simulink model "Copy_of_modello_completo_2_12"  (R2020b)
settings: Solver=FixedStepDiscrete  StartTime=0.0  StopTime=Inf  FixedStep=0.02  RelTol=1e-3  EnableMultiTasking=on
undefined symbols (not defined in the file or in its folder): attuatore_Amax, attuatore_Amin, attuatore_Emax, attuatore_Emin, attuatore_Rmax, attuatore_Rmin, attuatore_Tmax, attuatore_Tmin, DiscIntNeverNeededParam, interventoA_05, interventoA_1, interventoE_05, interventoE_1, interventoT, inv_A, inv_comp_h, inv_E, inv_R, inv_T, K_AW_B_AP_quota, K_AW_B_becc, K_AW_B_imb, K_AW_B_roll, K_imb_inv, Kd_h_app, Kd_h_flare, Ki_AP_quota_select, Ki_AP_rotta, Ki_AP_vel, Ki_becch, Ki_h_app, Ki_h_cruise, Ki_h_flare, Ki_roll, Kp_AP_quota_hold_h, Kp_AP_quota_hold_l, Kp_AP_quota_select, Kp_AP_rotta, Kp_AP_vel, Kp_becch, Kp_comp_h, Kp_h_app_max, Kp_h_app_min, Kp_h_cruise, Kp_h_flare, Kp_imb, Kp_p, Kp_q, Kp_roll, Kp_Rotta_ATO, Newton, phi_max, phi_min, Raphson, safe_phi, safe_V, t_AP, theta_max, theta_min, time_alarm_SAFE ... (+5)
libraries: simulink_extras x41, arduinolib x26, pid_lib x8, svdutilitieslib x6, simulink x3, dspsigops x3, aerolibtransform2sys x2, aerolibtransform2 x2, cstblocks x1
(part 6 of 8)

== stateflow chart Copy_of_modello_completo_2_12/AUTOPILOTA/Subsystem1/Subsystem1/Chart1 ==
  state Allignment1
    du:
    maneuver_selector=1;
    landing_selector=0;
    trig_approach = 0;
    trig_flare = 0;
    approach_selector = 0;
  state Abort
    du:
    maneuver_selector=1;
    landing_selector=0;
    trig_approach = 0;
    trig_flare = 0;
    approach_selector = 0;
  state Allignment
    du:
    trig_flare = 0;
    approach_selector = 0;
    maneuver_selector=1;
    landing_selector=0;
    trig_approach = 0;
  state Approach
    du:
    trig_flare = 0;
    trig_approach = 1;
    approach_selector = 1;
    landing_selector=1;
    maneuver_selector=2;
  state Flare
    du:
    trig_approach = 0;
    trig_flare = 1;
    approach_selector = 0;
    landing_selector=2;
    maneuver_selector=3;
  (default) -> Allignment1 : {maneuver_selector=1;
      |  landing_selector=0;
      |  trig_approach = 0;
      |  trig_flare = 0;
      |  approach_selector = 1;}
  Approach -> Allignment1 [order 2] : [modo ~= 4]
  Flare -> Allignment1 [order 2] : [modo ~= 4]
  Allignment -> Allignment1 [order 2] : [modo ~= 4]
  Approach -> Abort [order 3] : [landing_abort == 1]
  Allignment -> Approach [order 1] : [(h > 35) && (h < 60) && (dist <= h*(1/tan(3*pi/180))+100) && (dist >= h*(1/tan(4*pi/180))+100) && (counter >1)]
  Allignment1 -> Allignment : [modo == 4]
  Approach -> Flare [order 1] : [ (x_e >= x_f) && ((h <= (h_f + 1.5)) ||( h > (h_f - 1)))]
  Flare -> (junction 67) [order 1] : [TAS < 3]{landing_selector=0;}
  data: h input; dist input; counter input; maneuver_selector output; x_e input; x_f input; h_f input; TAS input; landing_selector output; trig_approach output; modo input; trig_flare output; approach_selector output; landing_abort input

== matlab function Copy_of_modello_completo_2_12/AIR TX/Heartbeat/Alarm set ==
  data: Alarm input; H_mav output; Rx_mode input

%%

function H_mav = Allarm_set(Alarm, Rx_mode)
%#cambia lo stato se c'è un allarme attivo
% Allarm: possibili allarmi proveniente dall'autopilota
% Rx_mode: richiesta da parte della stazione di terra
% H_mav: setto i parametri Base_mode e System_status del Heartbeat


H_mav = uint8(Rx_mode); % setta la modalità con quella ricevuta da terra

% se un allarme si attiva ha la precedenza sulla richiesta della QGC

if Alarm(1) == 1 % ovvero l'aereo è entrato in safe e si pone su traettoria circolare di sicurezza
    
    H_mav(1) = uint8(220); % MAV_MODE_AUTO_ARMED
    H_mav(2) = uint8(5);   % MAV_STATE_CRITICAL
%     H_mav(3) = uint8(128); % MAV_MODE_FLAG_SAFETY_ARMED

end

% se l'allareme di intervento pilota è attivo ha precedenza sull'allarm
% sefe per cui bisogna riscrivere lo stato del pilota

if Alarm(2) == 1 % si è attivato l'allarme dell'intervento pilota 
    
    H_mav(1) = uint8(216); % MAV_MODE_GUIDED_ARMED
    H_mav(2) = uint8(4);   % MAV_STATE_ACTIVE
%     H_mav(3) = uint8(8);   % MAV_MODE_FLAG_GUIDED_ENABLED

end

== matlab function Copy_of_modello_completo_2_12/AIR TX/If_subsystem/iflogic_function ==
  data: H50 input; iflogic output; H10 input
function iflogic = fcn(H50,H10)
%#codegen
% prende in ingeresso i counter che contano il tempo
% e dice quale messaggio bisogna inviare in base alle frequenze scelte in
% Heartbeat:            1Hz
% SCALED_IMU:           20Hz
%attitude:              20Hz
%GLOBAL_POSITION_INT:   1Hz
%SYS_STATUS:            3Hz
%VFR_HUD:               2Hz
%SERVO_OUTPUT_RAW       1Hz
%SCALED_PRESSURE        1Hz

if H50 == 1  || H50==3
    iflogic=uint8(26); % SCALED_IMU 20Hz
elseif H50==2 || H50==4
    iflogic=uint8(30); %attitude 20Hz
elseif  H50==0 && H10==2
    iflogic=uint8(33); %GLOBAL_POSITION_INT 1Hz
elseif  H50==0 && H10==6
    iflogic=uint8(34); %GLOBAL_POSITION_INT_RAW 1Hz
elseif  H50==0 && H10==0
    iflogic=uint8(0); %Heartbeat 1Hz
elseif H50==0 && (H10==1 || H10==5 || H10==9)
    iflogic=uint8(1); %SYS_STATUS 3Hz
elseif H50==0 && (H10==3 || H10==8)
    iflogic=uint8(74); %VFR_HUD 2Hz
elseif H50==0 && (H10==7)
    iflogic=uint8(36); %SERVO_OUTPUT_RAW 1Hz
elseif H50==0 && (H10==4)
    iflogic=uint8(29); %SCALED_PRESSURE 1Hz
else
    iflogic=uint8(255); %non esiste nessun messaggio con questo codice
    
end

== matlab function Copy_of_modello_completo_2_12/AIR TX/Waypoints/MATLAB Function ==
  data: WP_info_in input; WP_param_in input; WP_info output; GC_info input; WP_param output
function [WP_info,WP_param] = fcn(WP_info_in,WP_param_in, GC_info)
%#codegen
WP_info=WP_info_in(1,:); %%per sicurezza
WP_param=WP_param_in(1,:); %%per sicurezza
[m,n]=size(WP_info_in);
if GC_info(1)==2
    if GC_info(2)>=0 && GC_info(2)<m %per poter inviare i MISSION_ITEM
        WP_info=WP_info_in(GC_info(2)+1,:);
        WP_param=WP_param_in(GC_info(2)+1,:);
    end
end
if GC_info(1)==3 && GC_info(2)>=0 && GC_info(2)<200 %per poter inviae i MISSION_REQUEST
    WP_info=WP_info_in(GC_info(2)+1,:);
end

== matlab function Copy_of_modello_completo_2_12/AUTOPILOTA/Subsystem1/Subsystem/VETTORIALE ==
  data: V_vett output double; h_vett output double; rotta_vett output double; RC_vett output double; ingaggio_AP_mem output; modo input; IAS input; ALT input; HDG input; I_RC input; ingaggio_AP input; ROTTA input; VELOCITA input; QUOTA input; RC input; HEADING input; TAS input; h input; RC_default input; ingaggio_AP_pre input uint8; modo_pre input; IAS_pre input uint8; ALT_pre input uint8; HDG_pre input uint8; modo_pre_mem output; IAS_pre_mem output uint8; ALT_pre_mem output uint8; HDG_pre_mem output uint8
function [V_vett, h_vett, rotta_vett, RC_vett, ingaggio_AP_mem, modo_pre_mem, IAS_pre_mem, ALT_pre_mem, HDG_pre_mem] = vettoriale(modo, IAS, ALT, HDG, I_RC, ingaggio_AP ,ROTTA, VELOCITA, QUOTA, RC, HEADING, TAS, h, RC_default, ingaggio_AP_pre,modo_pre, IAS_pre, ALT_pre, HDG_pre)
%#codegen

persistent V_ref ALT_ref HDG_ref

if isempty(V_ref)
    
    V_ref = 0;
    
end

if isempty(ALT_ref)
    
    ALT_ref = 0;
    
end

if isempty(HDG_ref)
    
    HDG_ref = 0;
    
end

if (ingaggio_AP ~= ingaggio_AP_pre || modo ~= modo_pre || IAS ~= IAS_pre)
    
    V_ref = TAS;
    
end

if (ingaggio_AP ~= ingaggio_AP_pre || modo ~= modo_pre || ALT ~= ALT_pre)
    
    ALT_ref = h;
    
end

if (ingaggio_AP ~= ingaggio_AP_pre || modo ~= modo_pre || HDG ~= HDG_pre)
    
    HDG_ref = HEADING;
    
end

if (IAS == 1)
    
    V_vett = VELOCITA;
    
else
    
    V_vett = V_ref;
    
end

if (ALT == 1)
    
    h_vett = QUOTA;
    
else
    
   h_vett = ALT_ref;
    
end

if (HDG == 1)
    
    rotta_vett = ROTTA;
    
else
    
  rotta_vett = HDG_ref;
    
end

RC_vett = 0;

if ((h_vett - h) >= 0) 
    
    if (I_RC == 1)
    
        RC_vett = RC;
    
    else
    
        RC_vett = RC_default;
    
    end
    
elseif ((h_vett - h) < 0 ) 
    
    if (I_RC == 1)
    
        RC_vett = -RC;
    
    else
    
        RC_vett = -RC_default;
    
    end 
    
end
    
ingaggio_AP_mem = uint8(ingaggio_AP);
modo_pre_mem = modo;
IAS_pre_mem  = uint8(IAS);
ALT_pre_mem  = uint8(ALT);
HDG_pre_mem  = uint8(HDG);

== matlab function Copy_of_modello_completo_2_12/Misure Sensori/BMP_280/MATLAB Function1 ==
  data: T_0 input; P_ref input; h_ output; P input
function h_  = fcn( T_0, P_ref,P)
%#codegen

g     = 9.81;    %accelerazione di gravità
R_gas = 287.05;  %costante dei gas perfetti
dTdh  = -0.0065; %gradiente termico verticale in atmosfera standard 

T_0        = T_0+273.15;


    
h_= ((R_gas/g)*log(P_ref/P)*T_0)/(1-(dTdh*0.5*(R_gas/g)*log(P_ref/P)));

== matlab function Copy_of_modello_completo_2_12/AIR RX/MATLAB Function1 ==
  data: Base_mode input; GC_req input; value_c input; WP_info_in input; WP_param_in input; mem_out input; T_number input; T_ref input; Mav_state input; AP_int output; AP_rif output; H_mav output; SyS_data output; GC_info output; WP_db_out output; WP_db_param output; WP_AL output; Val_out_MAV output; T_0 output; AP_int_mem input; Base_mode_to_SF output; test output
function [AP_int, AP_rif, H_mav, SyS_data, GC_info, WP_db_out, WP_db_param,WP_AL, Val_out_MAV, T_0, Base_mode_to_SF, test] =...
    RXelaborazione(Base_mode, GC_req, value_c, WP_info_in, WP_param_in, mem_out, T_number, T_ref, Mav_state, AP_int_mem)
%#codegen
% PARTE PER LA GESTIONE DELLE RICHIESTE DALLA STAZIONE DI TERRA
% GC_req= richiesta della stazione di terra, vettore 2 componenti
%           GC_req(1)=1 :    inviare i parametri a fronte della ricezione del
%                           SET_Request
%                             se GC_req(2)=255 li invia tutti altrimenti
%                             solo 1
% value_c= valore da aggiornare;
% GC_info= necessario per S-function mavlink di trasmissione dipende dal
%               GC_req ricevuto
% WP_db_info= [WP_item255.count,WP_item255.seq,WP_item255.command,WP_item255.frame,
%               WP_item255.current,WP_info[5]=WP_item255.autocontinue]
% WP_db_param= parametri ultimo wp arrivato
% Val_out_MAV= valori aggiornati in uscita per il mavlink di trasmissione
% 
%  mem_out=[msg.sysid; msg.compid;msg.msgid;msg.len;msg.seq;flag]
%
% PARTE PER LA GESTIONE MANUALE AUTOMATICO
%Base_mode: richiesta da parte della stazione di terra di settare una
%           modalità di volo
%H_mav: setto i parametri Base_mode e System_status del Heartbeat di
%           trasmissione
%
%  VARIABILI NECESSARIE ALL'AUTOPILOTA
%AP_interruttori: interruttore di pilota automatico e manuale e modalità
%            [ manuale automatico HDG IAS ALT RC]
%
%AP_riferimenti: valori delle modalità di volo [HDG IAS ALT RC]

persistent riferimenti   % riferimenti delle modalità di volo
persistent WP_dbP WP_dbI WP_dbP_AL % lista dei parametri dei waypoint
persistent test1

nWPmax = uint16(6); % Numero massimo di WP da memorizzare %[MILONE]

% Inizializzazione

if isempty(riferimenti)
    
    riferimenti = single([0; 0; 0; 0; 0; 0; 0; 0; 20; 100; 2; 101325; 15; 0; 0; 0]) ; %valori di riferimento di ["I_HDG", "I_IAS", "I_ALT", "I_RC", "I_WP", "I_ATO", "I_AL" "V_HDG","V_IAS","V_ALT","V_RC","C_P0","C_T0","H_LAT","H_LONG","H_ALT"};]
    
end

if isempty(WP_dbP) || (GC_req(1) == 3 && GC_req(2) == 250)
    
        WP_dbP = single(zeros(nWPmax,7)); % nWPmax righe e 7 colonne
        WP_dbI = uint16(zeros(nWPmax,6)); % nWPmax righe e 6 colonne
        
        
end
if isempty(WP_dbP_AL) || (GC_req(1) == 3 && GC_req(2) == 250)                % introdotto da Sensolini: consente di inviare contemporaneamente wp di navigazione ed atterraggio
    
        WP_dbP_AL = single(zeros(nWPmax,7)); % nWPmax righe e 7 colonne
              
end

if isempty(test1)
    
    test1 = 0;
    
end


%% Parte di richieste da mavlik relativa al messaggio PARAM_SET

GC_info = [GC_req; mem_out(1)]; % GC_req (vettore di due) sarebbe GC_request nella S-Function ed è usato per la funzione di PARAM_SET; 
                                % mem_out(1) sarebbe nella S-Function mem_out[0]=msg.sysid; cioè chi interroga

if GC_info(1) == 1
    
    if GC_info(2) > 0 && GC_info(2) <= 7
        
        if abs(value_c) > 0 % attiva l'interruttore
            
            riferimenti(GC_info(2)) = single(1);
            
            %NB: se arrivano valori maggiori di 1 sempre 1 da in output perchè
            % gli interruttori possono essere solo di tipo 0/1
            % altrimenti l'autopilota si blocca
            
        elseif value_c == 0 % disattiva l'interruttore
            
            riferimenti(GC_info(2)) = single(0);
            
        end
        
    elseif GC_info(2) > 7 && GC_info(2) < 12
        
        riferimenti(GC_info(2)) = single(value_c);
        
    end
    
end

%% Parte relativa al messaggio COMMAND_LONG per la temperatura di riferimento dell'altimetro

if T_number == 13;
    
        riferimenti(T_number) = T_ref;
        
end

%%

Val_out_MAV = riferimenti; % output riferimenti

%% WP set

if GC_info(1) == 3 && GC_info(2) == 200 % arriva il numero dei waypoint
    
     if WP_info_in(1) > nWPmax  %%%ATTENZIONE!!  %[MILONE]
        WP_info_in(1) = nWPmax; % se nWP>nWPmax mi comporto come se avessi ricevuto solo i primi nWPmax
                                % non è ottimale, infatti QGC deve aspettare il time out, ma funziona
                                % va migliorata con una opportuna segnalazione
     end
     
     WP_dbI(:,1) = WP_info_in(1);
     
end

if GC_info(1) == 3 && GC_info(2) < 200 % è arrivato un waypoint
    
    if WP_param_in(2) == 0
    
    WP_dbP(WP_info_in(2)+1,:)   = single(WP_param_in); % 7Parametri. è arrivato il numero WP_info(2) +1 perchè in C si parte da 0
    WP_dbI(WP_info_in(2)+1,2:7) = WP_info_in(2:7);     % 6informazioni. è arrivato il numero WP_info(2)  +1 perchè in C si parte da 0
    
    else
     WP_dbP_AL(WP_param_in(1)+1,:) = single(WP_param_in);
     WP_dbI(WP_info_in(2)+1,2:7) = WP_info_in(2:7);
     
    end
    
end

WP_db_out   = WP_dbI;

WP_db_param = WP_dbP;
WP_AL = WP_dbP_AL;

%for i=1:WP_info_in(1)
%if WP_dbP(WP_info_in(2)+1,2) == 0
%    WP_db_param = WP_dbP;
%    WP_AL = single(zeros(nWPmax,7));
%else
%    WP_db_param = single(zeros(nWPmax,7));
%    WP_AL = WP_dbP;
%end
%end
%% parte di gestione modalità autopilota

H_mav   = uint8(zeros(2,1)); % inizializzo il vettore di output
AP_mode = uint8([0;0]);      % inizializzo il vettore che gli interrutori manuale e automatico

Base_mode_to_SF = uint8(0);

% setto i parametri necessari per l'hearbeat e per l'autopilota

if Base_mode == uint8(0) && Mav_state == uint8(0) % INIZIO: è la condizione che si verifica quando connetto Arduino a QGC, ovvero l'autopilota è in stato Standby
    
    H_mav(1) = uint8(0);         % MAV_MODE_PREFLIGHT
    H_mav(2) = uint8(3);         % MAV_STATE_STANDBY
%     H_mav(3) = uint8(64);        % MAV_MODE_FLAG_MANUAL_INPUT_ENABLED   %% il MAV_MODE_FLAG è commentato perché non lo utilizziamo dato che inviamo nel messaggio dell'heartbeat il MAV_MODE in corrispondenza del valore di base_mode (vedere la pagina web MAV'RIC)
    AP_mode  = uint8([1; 0]);    % attivo il manuale  spengo l'automatico
    Base_mode_to_SF = uint8(0);

elseif Base_mode == uint8(0) && Mav_state == uint8(3) % è arrivato MAV_MODE_PREFLIGHT e MAV_STATE_STANDBY (modalità Ready)
    
    H_mav(1) = uint8(0);         % MAV_MODE_PREFLIGHT
    H_mav(2) = uint8(3);         % MAV_STATE_STANDBY
%     H_mav(3) = uint8(64);        % MAV_MODE_FLAG_MANUAL_INPUT_ENABLED 
    AP_mode  = uint8([1; 0]);    % attivo il manuale  spengo l'automatico
    Base_mode_to_SF = uint8(0);
    test1 = 0;

elseif Base_mode == uint8(0) && Mav_state == uint8(2) % è arrivato MAV_MODE_PREFLIGHT e MAV_STATE_CALIBRATING
    
    H_mav(1) = uint8(0);         % MAV_MODE_PREFLIGHT
    H_mav(2) = uint8(2);         % MAV_STATE_CALIBRATING
%     H_mav(3) = uint8(64);        % MAV_MODE_FLAG_MANUAL_INPUT_ENABLED
    AP_mode  = uint8([1; 0]);    % attivo il manuale  spengo l'automatico
    Base_mode_to_SF = uint8(0);
    test1 = 0;
    
elseif Base_mode == uint8(0) && Mav_state == uint8(1) % è arrivato MAV_MODE_PREFLIGHT e MAV_STATE_BOOT
    
    H_mav(1) = uint8(0);         % MAV_MODE_PREFLIGHT
    H_mav(2) = uint8(1);         % MAV_STATE_BOOT
%     H_mav(3) = uint8(64);        % MAV_MODE_FLAG_MANUAL_INPUT_ENABLED
    AP_mode  = uint8([0; 1]);    % In questo caso si attiva l'interrutore di modalità automatica. 
                                 % Il motivo è dovuto al fatto che per fare la prova del safe è necessario che sia attivo 
                                 % il modo automatico altrimenti il safe non entra.
    Base_mode_to_SF = uint8(0);
    test1 = 1;
    
% elseif Base_mode==uint8(80)  %è arrivato MAV_MODE_STABILIZE_DISARMED, 1 manual in QGC
%     H_mav(1)=uint8(80);        %MAV_MODE_GUIDED_ARMED
%     H_mav(2)=uint8(4);          %MAV_STATE_ACTIVE
%     AP_mode=uint8([1; 0]);      %attivo il manuale  spengo l'automatico

elseif Base_mode == uint8(192) % è arrivato MAV_MODE_MANUAL_ARMED
    
    H_mav(1) = uint8(192);       % MAV_MODE_MANUAL_ARMED 
    H_mav(2) = uint8(4);         % MAV_STATE_ACTIVE
%     H_mav(3) = uint8(64);        % MAV_MODE_FLAG_MANUAL_INPUT_ENABLED
    AP_mode  = uint8([1; 0]);    % attivo il manuale  spengo l'automatico
    Base_mode_to_SF = uint8(192);
    
elseif Base_mode == uint8(208) % è arrivato MAV_MODE_STABILIZE_ARMED (sarebbe la modalità Stand By presente nello State Flow degli stati)
    
    H_mav(1) = uint8(208);       % MAV_MODE_STABILIZE_ARMED
    H_mav(2) = uint8(3);         % MAV_STATE_STANDBY
%     H_mav(3) = uint8(64);        % MAV_MODE_FLAG_MANUAL_INPUT_ENABLED
    AP_mode  = uint8([0; 0]);    % disattiva l'interruttore del manuale ma l'automatico non è ancora attivo
    Base_mode_to_SF = uint8(208);

elseif Base_mode == uint8(220) && Mav_state ~= uint8(5) % è arrivato MAV_MODE_AUTO_ARMED
    
    if (AP_int_mem(1) == uint8(0) && AP_int_mem(2) == uint8(0) && ((AP_int_mem(3) == uint8(1) || AP_int_mem(4) == uint8(1) ||...
        AP_int_mem(5) == uint8(1) || AP_int_mem(6) == uint8(1) || AP_int_mem(7) == uint8(1) || AP_int_mem(8) == uint8(1))))
    
        H_mav(1) = uint8(220);       % MAV_MODE_AUTO_ARMED
        H_mav(2) = uint8(4);         % MAV_STATE_ACTIVE
%         H_mav(3) = uint8(4);         % MAV_MODE_FLAG_AUTO_ENABLED
        AP_mode  = uint8([0; 1]);    % spengo il manuale attivo l'automatico
        Base_mode_to_SF = uint8(220);
        
    elseif (AP_int_mem(1) == uint8(0) && AP_int_mem(2) == uint8(1) && ((AP_int_mem(3) == uint8(1) || AP_int_mem(4) == uint8(1) ||...
            AP_int_mem(5) == uint8(1) || AP_int_mem(6) == uint8(1) || AP_int_mem(7) == uint8(1) || AP_int_mem(8) == uint8(1)))) 
        
        H_mav(1) = uint8(220);       % MAV_MODE_AUTO_ARMED
        H_mav(2) = uint8(4);         % MAV_STATE_ACTIVE
        AP_mode  = uint8([0; 1]);    % spengo il manuale attivo l'automatico
        Base_mode_to_SF = uint8(220);
        
    else 
        
        H_mav(1)  = uint8(208);       % MAV_MODE_STABILIZE_ARMED
        H_mav(2)  = uint8(3);         % MAV_STATE_STANDBY
        AP_mode   = uint8([0; 0]);    % attivo il manuale  spengo l'automatico
        Base_mode_to_SF = uint8(208);
    
    end

% elseif Base_mode == uint8(216)  % è arrivato MAV_MODE_GUIDED_ARMED
%     
%     H_mav(1) = uint8(8);         % MAV_MODE_FLAG_GUIDED_ENABLED
%     H_mav(2) = uint8(4);         % MAV_STATE_ACTIVE
%     AP_mode  = uint8([0; 1]);    % spengo il manuale attivo l'automatico
    
elseif Mav_state == uint8(5)  % si verifica nell'S-Function di ricezione quando il velivolo è andato in safe ovvero quando Alarm_Safe = 1
    
    H_mav(1) = uint8(220);      % MAV_MODE_AUTO_ARMED
    H_mav(2) = uint8(5);        % MAV_STATE_CRITICAL
%     H_mav(3) = uint8(128);      % MAV_MODE_FLAG_SAFETY_ARMED
    AP_mode  = uint8([0; 1]);   % spengo il manuale attivo l'automatico

% elseif Base_mode==uint8(66) % è arrivato MAV_MODE_TEST_DISARMED, lo usiamo per fare la calibrazione
%     H_mav(1)=uint8(64);        %MAV_MODE_FLAG_MANUAL_INPUT_ENABLED
%     H_mav(2)=uint8(2);         %MAV_STATE_CALIBRATING
%     AP_mode=uint8([1; 0]);     %attivo il manuale  spengo l'automatico
    
    %%%%%%%%%%%%%%%%%%%%%%%%%%%
    % elseif Base_mode==uint8(192) %%ARMED PREFLIGHT
    %     H_mav(1)=uint8(192);        %MAV_MODE_FLAG_MANUAL_INPUT_ENABLED
    %     H_mav(2)=uint8(3);          %	MAV_STATE_EMERGENCY
    %     AP_mode=uint8([0; 1]);     %spengo il manuale attivo l'automatico
    %     elseif Base_mode==uint8(64) %%DISARMED PREFLIGHT
    %     H_mav(1)=uint8(64);        %MAV_MODE_FLAG_MANUAL_INPUT_ENABLED
    %     H_mav(2)=uint8(3);          %	MAV_STATE_EMERGENCY
    %     AP_mode=uint8([0; 1]);     %spengo il manuale attivo l'automatico
    %     %%%%%%%%%%%%%%%%%%%%%%%%%%%%%%%%%%%%%%%

else
    
    H_mav(1) = uint8(192);       % MAV_MODE_MANUAL_ARMED 
    H_mav(2) = uint8(6);         % MAV_STATE_EMERGENCY
%     H_mav(3) = uint8(64);        % MAV_MODE_FLAG_MANUAL_INPUT_ENABLED
    AP_mode  = uint8([1; 0]);    % attivo il manuale  spengo l'automatico
    
end

%% parte delle informazioni sullo stato del sistema in ricezione

% calcolo dei messaggi persi provenienti dalla stazione di terra

drop_rate = 10*((100*mem_out(6))/mem_out(5));  % 10*percentuale !non moltipilicare direttamente per 10000 perchè è un uint16 e va in overflow
SyS_data  = [drop_rate mem_out(7) mem_out(3)];

%% parte per settare gli interrutori e i riferimenti

AP_int = [AP_mode; uint8(riferimenti(1:7))]; % interruttori
AP_rif = riferimenti(8:11);                  % riferimenti

T_0 = riferimenti(13); % valore della temperatura di riferimento T_0 dell'altimetro

test = test1;

== matlab function Copy_of_modello_completo_2_12/AIR RX/MATLAB Function4 ==
  data: byte_pack input; status output; messaggio output; messaggio_2 output; byte_available input
function [status,messaggio,messaggio_2]  = Creazione_mavlink_message_2(byte_pack,byte_available)


persistent Interr_parz  message counter len_found mess_len

if isempty(Interr_parz)
    Interr_parz = false ;
end
if isempty(message)
     message = uint8(zeros(1,100 )) ;
end
if isempty (counter) 
    counter = uint8(0) ;    % variabile che conta quanti byte mancano per completare il messaggio
end 

if isempty(len_found) 
     len_found = false ;
end 

if isempty(mess_len) 
     mess_len = 0 ;
end 

status = 0;
M = length(byte_pack) ;
caso = 0 ;
messaggio = uint8(zeros(1,100 )) ;
messaggio_2 = uint8(zeros(1,100 )) ;
% LA VARIABILE INTERR_PARZ va attivata a 1 alla fine della funzone di
% lettura per indicare di leggere il successivo messaggio in arrivo 

[poss_254,num_254] = find_254(byte_pack) ;

if ((Interr_parz == true) && (num_254 == 1))                  % in questo caso verifico che il 254 sia effettivamente un altro inizio
if (poss_254(1) ~= counter+1)
   num_254 = 0; 
end
    
end



if ( num_254 == 1 && Interr_parz == false )             
    caso = 1 ;                                                            % 1 Messaggio Intero   o parziale che inizia                % attivare alla fine della funzione Interr_parz == true o false 
elseif (num_254 == 0 && Interr_parz == true )
    caso = 2 ;                                                        % 1 Messaggio Parziale senza inizio e poi nulla 
elseif (num_254 == 1 && Interr_parz == true )                         
    caso = 3 ;                                                        % 1 Messaggio Parziale e poi un altro messaggio completo o parziale
elseif  ( num_254 == 2 && Interr_parz == false ) 
    caso = 4 ;                                                         % Due messaggi completi  oppure 1 Completo + parziale ( attivare Interr_parz alla fine del codice)
end


switch (caso)
   
    
    
    case 1 
        pos_254 = poss_254(num_254) ;
        
        if pos_254 == M                                                                          % se il 254 sta alla fine 
             message(1) = byte_pack(pos_254)  ;
            len_found = false ;
            Interr_parz = true ;
        else
             len = byte_pack(pos_254 + 1)  ;
             if len <= 100
             if  ((byte_pack(poss_254(1)+1) + 8) == byte_available)                                             % se abbiamo tutto il messaggio all'interno del byte_pack
                message(1: 8 + len ) = byte_pack(pos_254 : pos_254 + (7+len) ) ;          % era cosi byte_pack(pos_254 : pos_254 + (8+len) ) ;
                messaggio = message ;
                status = 1 ;
                message = uint8(zeros(1,100 )) ;
                counter = uint8(0) ;
                len_found = true ;
                mess_len = 0 ;
             elseif ((byte_pack(poss_254(1)+1) + 8) > byte_available)
                mess_len = double(byte_available) ;                                       % lunghezza del messaggio da leggere dal byte_pack ( non uguale alla lunghezza del messaggio complessivo)
                message(1 : mess_len) = byte_pack(pos_254 : mess_len ) ;
                len_found = true ;
                counter = 8 + len - mess_len ;
                Interr_parz = true ;
             end
             else
                 messaggio = uint8(zeros(1,100 )) ;              
                 Interr_parz = false;
                 message = uint8(zeros(1,100 )) ;
                 counter = uint8(0) ;
                 len_found = false ;
                 mess_len = 0 ; 
                 status = 1 ;
             end   
             
        end
        
        
        
        
    case 2 
        
                                     % se la lunghezza è stata trovata e quindi ho il valore di counter che indica quante componenti mancano
           if byte_pack ~= 0
                message(mess_len + 1 : mess_len + counter) = byte_pack( 1 : counter) ;
                Interr_parz = false ;
                messaggio = message ;
                status = 1 ;
                message = uint8(zeros(1,100 )) ;
                len_found = true ;
                mess_len = 0 ;
                counter = uint8(0) ;
                
           else                                                    % se ho un messaggio parziale e nello step successivo non ricevo nulla allora azzero tutto, altrimenti entro in un loop infinito di messaggi sbagliati
                Interr_parz = false ;
                messaggio = uint8(zeros(1,100)) ;
                status = 1 ;
                message = uint8(zeros(1,100 )) ;
                len_found = true ;
                mess_len = 0 ;
                counter = uint8(0) ;  
           end        
        
        

  
        
    case 3 
        
                                     % se la lunghezza è stata trovata e quindi ho il valore di counter che indica quante componenti mancano
        pos_254 = poss_254(num_254) ;
        
                message(mess_len + 1 : mess_len + counter) = byte_pack( 1 : counter) ;
                Interr_parz = false ;
                messaggio = message ;
                status = 1 ;
                message = uint8(zeros(1,100 )) ;
                len_found = true ;
                mess_len = 0 ;
                counter = uint8(0) ;
                
             len = byte_pack(pos_254 + 1)  ;
             if len <= 100
             if  ((byte_pack(poss_254(1)+1) + 8) == uint8(byte_available-double(counter)))                                             % se abbiamo tutto il messaggio all'interno del byte_pack
                message(1: 8 + len ) = byte_pack(pos_254 : pos_254 + (7+len) ) ;          % era cosi byte_pack(pos_254 : pos_254 + (8+len) ) ;
                messaggio_2 = message ;
                status = 1 ;
                message = uint8(zeros(1,100 )) ;
                counter = uint8(0) ;
                len_found = true ;
                mess_len = 0 ;
             elseif ((byte_pack(poss_254(1)+1) + 8) > (uint8(byte_available)-counter))
                mess_len = double(byte_available) - double(counter) ;                                       % lunghezza del messaggio da leggere dal byte_pack ( non uguale alla lunghezza del messaggio complessivo)
                message(1 : mess_len) = byte_pack(pos_254 : mess_len ) ;
                len_found = true ;
                counter = 8 + len - mess_len ;
                Interr_parz = true ;
             end
             else
                 messaggio = uint8(zeros(1,100 )) ;              
                 Interr_parz = false;
                 message = uint8(zeros(1,100 )) ;
                 counter = uint8(0) ;
                 len_found = false ;
                 mess_len = 0 ; 
                 status = 1 ;
             end
                
      
            
        
        
        
      
        
        
    case 4
        primo_254 = poss_254(1) ;
        secondo_254 = poss_254(2) ;
        len_primo = byte_pack(primo_254 + 1) ;
    %    messaggio(1 : len_primo + 8) = byte_pack(primo_254 : primo_254 + (len_primo + 7)) ;           %era cosi      byte_pack(primo_254 : secondo_254 - 1)  ;

        if len_primo <= 100
        messaggio(1 : len_primo + 8) = byte_pack(primo_254 : primo_254 + (len_primo + 7)) ;             %era cosi      byte_pack(primo_254 : secondo_254 - 1)  ;
        else
        messaggio = uint8(zeros(1,100 )) ;
        Interr_parz = false;
        message = uint8(zeros(1,100 )) ;
        counter = uint8(0) ;
        len_found = false ;
        mess_len = 0 ;
        end
        
        status = 1;
        
             len = byte_pack(secondo_254 + 1)  ;
             if (len <= 100 && (secondo_254-primo_254 > 3))
             if ( (byte_available - ( secondo_254))  == 7 + len    )                                         % se abbiamo tutto il messaggio all'interno del byte_pack
                message(1: 8 + len ) = byte_pack(secondo_254 : secondo_254 + (7+len) ) ;      % era cosi byte_pack(pos_254 : pos_254 + (8+len) ) ;
                messaggio_2 = message ;
                status = 2 ;
                message = uint8(zeros(1,100 )) ;
                counter = uint8(0) ;
                len_found = true ;
                mess_len = 0 ;
             else
                mess_len = length(byte_pack(secondo_254:byte_available ) ) ;    % lunghezza del messaggio da leggere dal byte_pack ( non uguale alla lunghezza del messaggio complessivo)
                message(1 : mess_len) = byte_pack(secondo_254:byte_available ) ;
                len_found = true ;
                counter = 8 + len - mess_len ;
                Interr_parz = true ;
             end
             else
               messaggio_2 = uint8(zeros(1,100 )) ;              
               Interr_parz = false;
               message = uint8(zeros(1,100 )) ;
               counter = uint8(0) ;
               len_found = false ;
               mess_len = 0 ;    
              end
             
        
        
end
end






function [position,counter] = find_254(pack) 
    position = zeros(1,3) ;
    
    M = length(pack)  ;   
    counter = 0 ;
    for i = 1 : M
        if pack(i) == 254 
            counter = counter + 1;  
            position(counter) = i; 
        end
    end
    l = pack(position(1)+1);
    if counter > 1
    if ((pack(l+8+position(1)) ~= 254) && (position(1) ~= 0))
        counter = 1;
        position(2) = 0;
    end
    end
end

== matlab function Copy_of_modello_completo_2_12/MISURE DA SENSORI FILTRATE/TX & RX Seriale Arduino Raspberry/Subsystem1/MATLAB Function1 ==
  data: byte_pack input; status output; check output; messaggio output; mess_prec input uint8
function [status,check,messaggio]  = LETTURA_Rasp_mex(byte_pack,mess_prec)


status = false;   
check = false;
messaggio = uint8(zeros(1,27)) ;
M = uint8(length(byte_pack)) ;



if ( (byte_pack(1) == 255) &&  (byte_pack(2) == 254) && (byte_pack(M) == 60))
    messaggio = byte_pack;
    status = true;
    check = false;
else
    messaggio = mess_prec;
    check = true;
    status = true;
end

== stateflow chart Copy_of_modello_completo_2_12/AUTOPILOTA/Subsystem1/Chart ==
  state AutoTakeoff
    Wp_selector = 0;
    Vec_selector = 0;
    Ato_selector = 1;
    Al_selector = 0;
    Go_home_selector = 0;
  state Waypoint
    Wp_selector = 1;
    Vec_selector = 0;
    Ato_selector = 0;
    Al_selector = 0;
    Go_home_selector = 0;
  state In
    Wp_selector = 0;
    Vec_selector = 0;
    Ato_selector = 0;
    Al_selector = 0;
    Go_home_selector = 0;
  state AutoLanding
    Wp_selector = 0;
    Vec_selector = 0;
    Ato_selector = 0;
    Al_selector = 1;
    Go_home_selector = 0;
  state Vettoriale
    Wp_selector = 0;
    Vec_selector = 1;
    Ato_selector = 0;
    Al_selector = 0;
    Go_home_selector = 0;
  state GoHome
    Wp_selector = 0;
    Vec_selector = 0;
    Ato_selector = 0;
    Al_selector = 0;
    Go_home_selector = 1;
  AutoTakeoff -> Waypoint [order 2] : [Ap_sel == 1 && modo == 1]
  Waypoint -> In [order 2] : [Ap_sel == 0]
  AutoTakeoff -> In [order 1] : [Ap_sel == 0]
  (default) -> In : {Wp_selector = 0;
      | Vec_selector = 0;
      | Ato_selector = 0;
      | Al_selector = 0;}
  Waypoint -> AutoLanding [order 4] : [Ap_sel == 1 && modo == 4]
  In -> Waypoint [order 1] : [Ap_sel == 1 && modo == 1]
  In -> AutoTakeoff [order 5] : [Ap_sel == 1 && modo == 3]
  AutoLanding -> Waypoint [order 3] : [Ap_sel == 1 && modo == 1]
  AutoLanding -> In [order 1] : [Ap_sel == 0]
  Vettoriale -> In [order 1] : [Ap_sel == 0]
  AutoTakeoff -> Vettoriale [order 3] : [Ap_sel == 1 && modo == 2]
  Waypoint -> GoHome [order 1] : [Ap_sel == 1&& modo == 5]
  Waypoint -> Vettoriale [order 3] : [Ap_sel == 1 && modo == 2]
  Vettoriale -> Waypoint [order 2] : [Ap_sel == 1 && modo == 1]
  In -> AutoLanding [order 4] : [Ap_sel == 1 && modo == 4]
  In -> GoHome [order 3] : [Ap_sel == 1 && modo == 5]
  GoHome -> In : [Ap_sel == 0]
  In -> Vettoriale [order 2] : [Ap_sel == 1 && modo == 2]
  Vettoriale -> AutoLanding [order 4] : [Ap_sel == 1 && modo == 4]
  AutoLanding -> Vettoriale [order 2] : [Ap_sel == 1 && modo == 2]
  AutoLanding -> GoHome [order 4] : [Ap_sel == 1 && modo == 5]
  Vettoriale -> GoHome [order 3] : [Ap_sel == 1&& modo == 5]
  data: Al_selector output; Ato_selector output; Go_home_selector output; Vec_selector output; Wp_selector output; modo input; Ap_sel input

== stateflow chart Copy_of_modello_completo_2_12/AUTOPILOTA/AUTOPILOTI1/CONTROLLORE DI QUOTA/SELEZIONE MODALITA' HOLD//SELECT ==
  state Select
    during:
    mod=1;
  state Hold
    during:
    mod=0;
  (default) -> Select
  Select -> Hold : [deltah<10]
  Hold -> Select : [deltah>10]
  data: mod output double; deltah input

== stateflow chart Copy_of_modello_completo_2_12/AUTOPILOTA/GESTIONE AUTOPILOTI1/ STATI ==
  state Go_Home
    during:
    modo = 5;
    switch_manetta = 1;
    switch_equilibratore =1;
    switch_alettoni=1;
    switch_timone=1;
  state MANUALE
    during:
    switch_manetta=0;
    switch_equilibratore=0;
    switch_alettoni=0;
    switch_timone=0;
  state Safe
    during:
    switch_manetta=1;
    switch_equilibratore=1;
    switch_alettoni=1;
    switch_timone=1;
    phi_safe=0.1745;
    theta_safe=0.05;
    throttle_safe=0.1;
  state Intervento_Pilota
    during:
    switch_manetta=0;
    switch_equilibratore=0;
    switch_alettoni=0;
    switch_timone=0;
  state AUTOMATICA
    state WAYPOINT
      during:
      modo = 1;
      switch_manetta = 1;
      switch_equilibratore =1;
      switch_alettoni=1;
      switch_timone=1;
    state TEST
      during:
      switch_manetta = 0;
      switch_equilibratore = 0;
      switch_alettoni = 0;
      switch_timone = 0;
    state VETTORIALE
      during:
      modo = 2;
      switch_manetta = 1;
      switch_equilibratore =1;
      switch_alettoni=1;
      switch_timone=1;
    state DECOLLO_AUTOMATICO
      during:
      modo = 3;
      switch_manetta = 1;
      switch_equilibratore = 1;
      switch_alettoni = 1;
      switch_timone = 1;
    state ATTERRAGGIO_AUTOMATICO
      during:
      modo = 4;
      switch_manetta = 1;
      switch_equilibratore =1;
      switch_alettoni=1;
      switch_timone=1;
    DECOLLO_AUTOMATICO -> WAYPOINT [order 2] : [WP_nav == 1 && h>30]
    TEST -> VETTORIALE : [test==0]
    WAYPOINT -> VETTORIALE [order 1] : [WP_nav == 0 &&  (IAS == 1 || ALT == 1 || HDG == 1||ATO==1)]
    (default) -> VETTORIALE
    VETTORIALE -> TEST [order 1] : [test==1]
    ATTERRAGGIO_AUTOMATICO -> WAYPOINT [order 1] : [AL==0 && h>20 && WP_nav==1 ]
    WAYPOINT -> ATTERRAGGIO_AUTOMATICO [order 2] : [AL==1]
    VETTORIALE -> WAYPOINT [order 4] : [WP_nav == 1]
    ATTERRAGGIO_AUTOMATICO -> VETTORIALE [order 2] : [AL==0 && h>20]
    DECOLLO_AUTOMATICO -> VETTORIALE [order 1] : [ATO == 0 && Tas >= 1 && (IAS == 1 || ALT == 1 || HDG == 1) ]
    VETTORIALE -> ATTERRAGGIO_AUTOMATICO [order 3] : [AL==1]
    VETTORIALE -> DECOLLO_AUTOMATICO [order 2] : [ATO == 1 && v_< 1]
    ATTERRAGGIO_AUTOMATICO -> DECOLLO_AUTOMATICO [order 3] : [ATO == 1 && AL == 0 && h<1 && v_<1]
  state Stand_By
    during:
    switch_manetta=0;
    switch_equilibratore=0;
    switch_alettoni=0;
    switch_timone=0;
  MANUALE -> Go_Home [order 1] : [Go_Home == 1 && Alarm_Safe == 0]
  Go_Home -> Intervento_Pilota [order 3] : [Alarm_Intervento==1]
  Go_Home -> Safe [order 2] : [Alarm_Safe == 1]
  (default) -> MANUALE
  AUTOMATICA -> Go_Home [order 3] : [Go_Home == 1]
  Go_Home -> AUTOMATICA [order 1] : [Go_Home == 0 && (WP_nav == 1 || IAS == 1 || ALT == 1 || HDG == 1|| AL == 1)]
  Safe -> MANUALE [order 2] : [MANUALE==1]
  Safe -> Intervento_Pilota [order 1] : [Alarm_Intervento==1]
  AUTOMATICA -> Safe [order 2] : [Alarm_Safe==1]
  Intervento_Pilota -> MANUALE : [MANUALE==1]
  AUTOMATICA -> Intervento_Pilota [order 1] : [Alarm_Intervento==1]
  AUTOMATICA -> MANUALE [order 5] : [MANUALE==1]
  Stand_By -> MANUALE [order 2] : [MANUALE==1]
  MANUALE -> Stand_By [order 2] : [MANUALE==0]
  Stand_By -> AUTOMATICA [order 1] : [Ingaggio_A_P==1]
  AUTOMATICA -> Stand_By [order 4] : [Ingaggio_A_P==0]
  data: MANUALE input; Ingaggio_A_P input; WP_nav input; ALT input; IAS input; HDG input; switch_manetta output double; switch_equilibratore output double; switch_alettoni output double; switch_timone output double; Alarm_Safe input; phi_safe output double; theta_safe output double; throttle_safe output double; Alarm_Intervento input; modo output double =1; ATO input; Tas input; AL input; v_ input; test input; h input; Go_Home input

== matlab function Copy_of_modello_completo_2_12/AUTOPILOTA/GESTIONE AUTOPILOTI1/Intervento Manager/MATLAB Function1 ==
  data: Manuale input; Int_1 output; sw output; Ingaggio_AP input; absE input; absA input; absT input; Int_05 output; interventoE_1 input; interventoE_05 input; interventoA_1 input; interventoA_05 input; interventoT input
function [Int_1, sw, Int_05] = Intervento(Manuale, Ingaggio_AP, absE, absA, absT, interventoE_1, interventoE_05, interventoA_1, interventoA_05, interventoT)
%#codegen

% persistent Ef Af Tf;
% 
% if (isempty(Ef) || Manuale == 1 || Ingaggio_AP == 0)
%     
%     Ef = absE;
%     Af = absA;
%     Tf = absT;   
%     
% end

persistent Tf;

if (isempty(Tf) || Manuale == 1 || Ingaggio_AP == 0)
    
    Tf = absT;  
    
end

if Ingaggio_AP == 1

%     dE = abs((Ef-absE));
%     dA = abs((Af-absA));
    dT = abs((Tf-absT));
    
%     if ((dE > 0.017 && dE < 0.1) && ALT == 1) % range compreso tra 0.97 e 5.73 deg di equilibratore

    if (absE > interventoE_1 && absE < interventoE_05) % interventoE_1 pari a 3.2 deg (il valore di trim dell'equilibratore alla massima velocità è di 3.18 deg)
                                                       % interventoE_05 pari al 30% (7.5 deg) del valore massimo assumibile dall'equilibratore pari a 25 deg.
                                                       % vedere il file Soglie_intervento.mat
        
        Int_1  = 1; % in questo caso scatta Int_temporiz il che significa che per attivarsi...  
        Int_05 = 0; % l'intervento pilota deve essere soddisfatta anche la successiva...
        sw            = 1; % condizione sul tempo di durata del comando sull'equilibratore 
                           
%     elseif (dE > 0.1 && ALT == 1)

    elseif absE > interventoE_05
        
        Int_1  = 0;
        Int_05 = 1;
        sw            = 0;
    
%     elseif ((dA > 0.017 && dA < 0.087) && HDG == 1) % range compreso tra 0.97 e 4.98 deg di alettoni

    elseif (absA > interventoA_1 && absA < interventoA_05) % interventoA_1 pari a 2 deg 
                                                           % interventoA_05 pari al 30% (6 deg) del valore massimo assumibile dall'alettone pari a 20 deg.

        Int_1  = 1;
        Int_05 = 0;
        sw            = 1;
        
%     elseif (dA > 0.087 && HDG == 1)

    elseif absA > interventoA_05
        
        Int_1  = 0;
        Int_05 = 1;
        sw            = 0;
   
    elseif dT > interventoT % interventoT uguale al 10% del valore massimo di manetta pari a 1; 0.1 sono circa tre scatti di comando della manetta
        
        Int_1  = 0; % nel caso della manetta se si supera la soglia scatta direttamente l'intervento pilota... 
        Int_05 = 1; % senza il controllo sul tempo
        sw            = 0;
        
    else
        
        Int_1  = 0;
        Int_05 = 0;
        sw            = 1;
                
    end
    
else
        
    Int_1  = 0; % quando il velivolo è in modo manuale gli interruttori sono posti a zero
    Int_05 = 0;
    sw            = 1;

end
    
end

== matlab function Copy_of_modello_completo_2_12/AUTOPILOTA/GESTIONE AUTOPILOTI1/MATLAB Function ==
  data: modo input; Switch_ATO output; Switch_AL output
function [Switch_ATO,Switch_AL] = fcn(modo)

persistent ATO AL

if modo == 3
    ATO = 1;
    AL = 0;
elseif modo == 4 
    AL = 1;
    ATO = 0;
else
    ATO = 0;
    AL = 0;
end

Switch_ATO = ATO;
Switch_AL = AL;

== matlab function Copy_of_modello_completo_2_12/AUTOPILOTA/GESTIONE AUTOPILOTI1/Safe Manager/MATLAB Function1 ==
  data: Veloc input; phi input; Alarm_safe output; ingaggio_AP input; safe_V input; safe_phi input; Manuale input
function Alarm_safe = fcn(Veloc, phi, ingaggio_AP, safe_V, safe_phi, Manuale)
%#codegen
persistent alarm;

if (isempty(alarm))
    
    alarm = 0;

end

if (ingaggio_AP == 1 && (Veloc > safe_V || abs(phi) > safe_phi)) % soglia sulla velocità impostata a 40 m/s e soglia sull'angolo di rollio impostata a 45 deg
    
    alarm = 1;  

elseif (Manuale == 1) % l'allarme si disattiva solo quando si entra in modalità Manuale
    
    alarm = 0;

end 

Alarm_safe = alarm;

end
